simulink model "modelGA"  (R2025b)
settings: Solver=FixedStepAuto  StartTime=0.0  StopTime=30  FixedStep=0.01  RelTol=1e-3
model workspace (MAT data in the model file):
  freq = 0.87
values from neighbouring files (symbols this model uses):
  A = [ 0        1         0        0 ... (first row only)    [gaOptimize.m]    (also in modelSetup.m)
  B = [0; 1/JD; 0; 0]    [gaOptimize.m]    (also in modelSetup.m = [0)
  C = [180/pi  0       0        0 ... (first row only)    [gaOptimize.m]    (also in modelSetup.m)
  D = zeros(4,1)    [gaOptimize.m]    (also in modelSetup.m = [0; 0; 0; 0])
  pwm = k * 125    [measureMotorDiff.m]    (also in modelSetup.m = 2000)
settings Model: Creator=marko  LastModifiedBy=Marko
settings DebuggingCC: UnconnectedInputMsg=warning  UnconnectedOutputMsg=warning  UnconnectedLineMsg=warning
settings ModelReferenceCC: EnableRefExpFcnMdlSchedulingChecks=on
settings RTWCC: GPUComputeCapability=3.5  DLArmComputeVersion=19.05

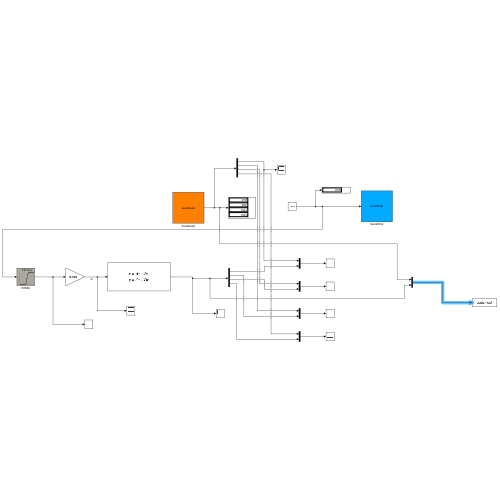
[thumbnail: Simulink's stored preview of the top-level diagram]
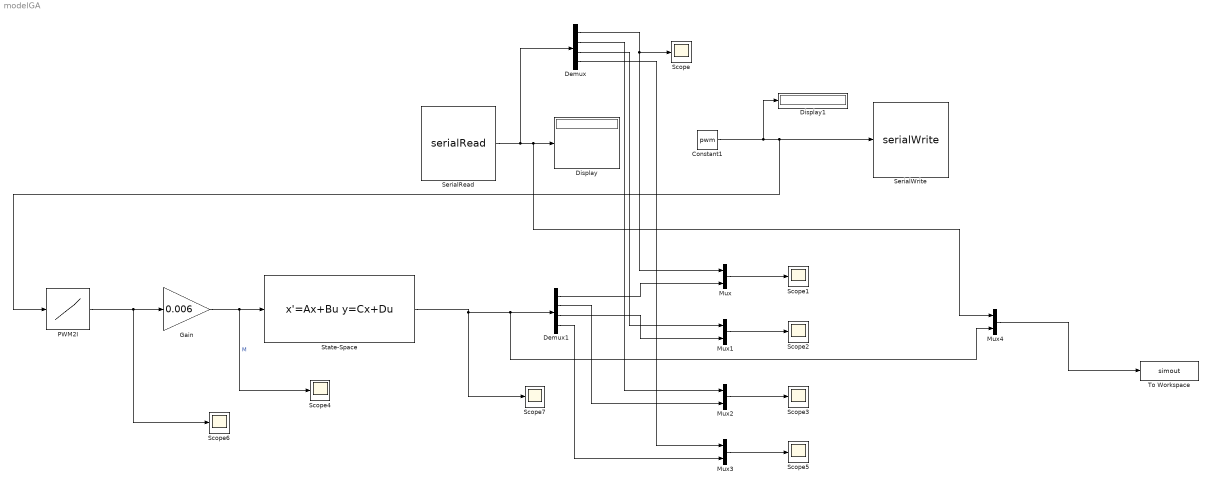
== system modelGA ==
  Constant1 : Constant  Value=pwm
  Demux : Demux
  Demux1 : Demux
  Display : Display
  Display1 : Display
  Gain : Gain  Gain=0.006
  Mux{,1..4} (5 alike) : Mux  Inputs=2
  PWM2I : Lookup_n-D  NumberOfTableDimensions=1  BreakpointsForDimension1=|  Table=|  InternalRulePriority=Speed  RndMeth=Simplest
      BreakpointsForDimension1=|
      | [ ...
      |    -4000; -3875; -3750; -3625; -3500; -3375; -3250; -3125; ...
      |    -3000; -2875; -2750; -2625; -2500; -2375; -2250; -2125; ...
      |    -2000; -1875; -1750; -1625; -1500; -1375; -1250; -1125; ...
      |    -1000;  -875;  -750;  -625;  -500;  -375;  -250;  -125; ...
      |        0; ...
      |      125;   250;   375;   500;   625;   750;   875;  1000; ...
      |     1125;  1250;  1375;  1500;  1625;  1750;  1875;  2000; ...
      |     2125;  2250;  2375;  2500;  2625;  2750;  2875;  3000; ...
      |     3125;  3250;  3375;  3500;  3625;  3750;  3875;  4000  ...
      | ]
      Table=|
      | [ ...
      |    -1.0346; -1.0331; -1.0334; -1.0337; -1.0310; -1.0314; -1.0297; -1.0293; ...
      |    -1.0298; -1.0276; -1.0263; -1.0253; -1.0241; -1.0237; -1.0225; -1.0194; ...
      |    -1.0188; -1.0142; -1.0117; -1.0059; -1.0031; -0.9984; -0.9934; -0.9842; ...
      |    -0.9693; -0.9515; -0.9373; -0.9088; -0.8800; -0.8097; -0.6768;  0.0000; ...
      |     0.0000; ...
      |     0.0000;  0.0000;  0.5970;  0.7090;  0.7996;  0.8580;  0.9030;  0.9253; ...
      |     0.9417;  0.9608;  0.9725;  0.9807;  0.9874;  0.9956;  1.0006;  1.0035; ...
      |     1.0095;  1.0121;  1.0126;  1.0158;  1.0181;  1.0181;  1.0185;  1.0202; ...
      |     1.0217;  1.0219;  1.0243;  1.0251;  1.0249;  1.0144;  1.0082;  1.0080  ...
      | ]
  Scope{,1..7} (8 alike) : Scope
      Scope settings: TimeSpan=500  ActiveDisplayYMinimum=-1  ActiveDisplayYMaximum=1
      Scope1 settings: TimeSpan=500  ActiveDisplayYMinimum=-419.71069337499989  ActiveDisplayYMaximum=3777.396240375
      Scope2 settings: TimeSpan=500  ActiveDisplayYMinimum=-159.149430425105  ActiveDisplayYMaximum=234.50498338056721  DataLoggingVariableName=ScopeData2
      Scope3 settings: TimeSpan=500  ActiveDisplayYMinimum=-1  ActiveDisplayYMaximum=1  DataLoggingVariableName=ScopeData3
      Scope4 settings: TimeSpan=500  ActiveDisplayYMinimum=9.3173750000000016E-6  ActiveDisplayYMaximum=2.9317375E-5  DataLoggingVariableName=ScopeData4
      Scope5 settings: TimeSpan=500  ActiveDisplayYMinimum=-1  ActiveDisplayYMaximum=1  DataLoggingVariableName=ScopeData5
      Scope6 settings: TimeSpan=500  ActiveDisplayYMinimum=0.25344768711381838  ActiveDisplayYMaximum=1.7458784803870731  DataLoggingVariableName=ScopeData6
      Scope7 settings: TimeSpan=500  ActiveDisplayYMinimum=-83.921597728546232  ActiveDisplayYMaximum=119.74437955691555  DataLoggingVariableName=ScopeData7
  SerialRead : M-S-Function  FunctionName=serialRead  Parameters='COM5'
  SerialWrite : M-S-Function  FunctionName=serialWrite  Parameters='COM5'
  State-Space : StateSpace  A=A  B=B  C=C  D=D  InitialCondition=0
  To Workspace : ToWorkspace  VariableName=simout  SaveFormat=Timeseries  SampleTime=-1
  wires:
  SerialRead/1 -> Demux/1, Mux4/1, Display/1
  Constant1/1 -> PWM2I/1, SerialWrite/1, Display1/1
  State-Space/1 -> Scope7/1, Mux4/2, Demux1/1
  Demux/1 -> Mux/1, Scope/1
  Gain/1 -> Scope4/1, State-Space/1  "M"
  PWM2I/1 -> Scope6/1, Gain/1
  Demux1/1 -> Mux/2
  Mux/1 -> Scope1/1
  Demux1/3 -> Mux1/2
  Demux/3 -> Mux1/1
  Mux1/1 -> Scope2/1
  Mux3/1 -> Scope5/1
  Mux2/1 -> Scope3/1
  Demux/2 -> Mux2/1
  Demux1/2 -> Mux2/2
  Demux/4 -> Mux3/1
  Demux1/4 -> Mux3/2
  Mux4/1 -> To Workspace/1
